simulink model "Ecuaciones_diferenciales"  (R2023b)
settings: Solver=VariableStepAuto  StartTime=0.0  StopTime=inf  RelTol=1e-3
InitFcn:
  | R = 52
  | L = 9.11 * 10^-9
  | K = 0.0593
  | J = 0.0632
  | b = 3.19 * 10^-9
settings Model: Creator=Carlos  LastModifiedBy=Carlos

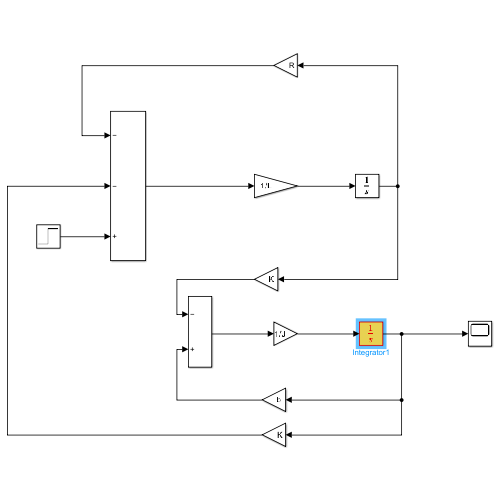
[thumbnail: Simulink's stored preview of the top-level diagram]
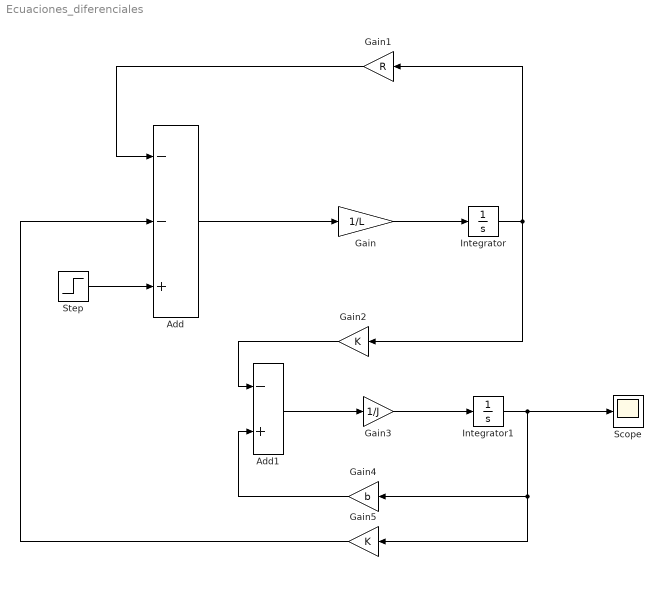
== system Ecuaciones_diferenciales ==
  Add : Sum  Inputs=--+
  Add1 : Sum  Inputs=-+
  Gain : Gain  Gain=1/L
  Gain1 : Gain  Gain=R
  Gain2 : Gain  Gain=K
  Gain3 : Gain  Gain=1/J
  Gain4 : Gain  Gain=b
  Gain5 : Gain  Gain=K
  Integrator : Integrator
  Integrator1 : Integrator
  Scope : Scope
  Step : Step  SampleTime=0
  wires:
  Add/1 -> Gain/1
  Gain/1 -> Integrator/1
  Integrator/1 -> Gain2/1, Gain1/1
  Gain1/1 -> Add/1
  Gain2/1 -> Add1/1
  Add1/1 -> Gain3/1
  Gain3/1 -> Integrator1/1
  Integrator1/1 -> Scope/1, Gain5/1, Gain4/1
  Gain4/1 -> Add1/2
  Gain5/1 -> Add/2
  Step/1 -> Add/3
